simulink model "MPC_regul_real"  (R2017a)
settings: Solver=VariableStepAuto  StartTime=0.0  StopTime=40  RelTol=1e-3
values from neighbouring files (symbols this model uses):
  P_0 = eye(8)*100    [MPC_setup_nonlinear.m]    (also in sim_phi_ref.mat = [100 0 0 0 0 0 0 0 0 100 0 0 ... (64 elements, 8x8)]; sim_theta_ref.mat = [100 0 0 0 0 0 0 0 0 100 0 0 ... (64 elements, 8x8)])
  R1 = sqrtm(R)    [MPC_setup_nonlinear.m]    (also in sim_phi_ref.mat = [0.00081901538426  9.06300190075e-05; 9.06300190075e-05  0.0; sim_theta_ref.mat = [0.00081901538426  9.06300190075e-05; 9.06300190075e-05  0.0)
  Ts_control = 0.05    [MPC_setup_nonlinear.m]    (also in sim_phi_ref.mat = 0.02; sim_theta_ref.mat = 0.02)
  Ts_kalman = 0.01    [MPC_setup_nonlinear.m]    (also in sim_phi_ref.mat; sim_theta_ref.mat)
  x_0 = [0,-pi/4,0,0,0,0,0,0]    [MPC_setup_nonlinear.m]    (also in sim_phi_ref.mat = [0 -0.785398163397 0 0 0 0 0 0]; sim_theta_ref.mat = [0 -0.785398163397 0 0 0 0 0 0])
settings Model: Creator=sverreknutsen  LastModifiedBy=sverreknutsen
settings SolverCC: AlgebraicLoopSolver=LineSearch

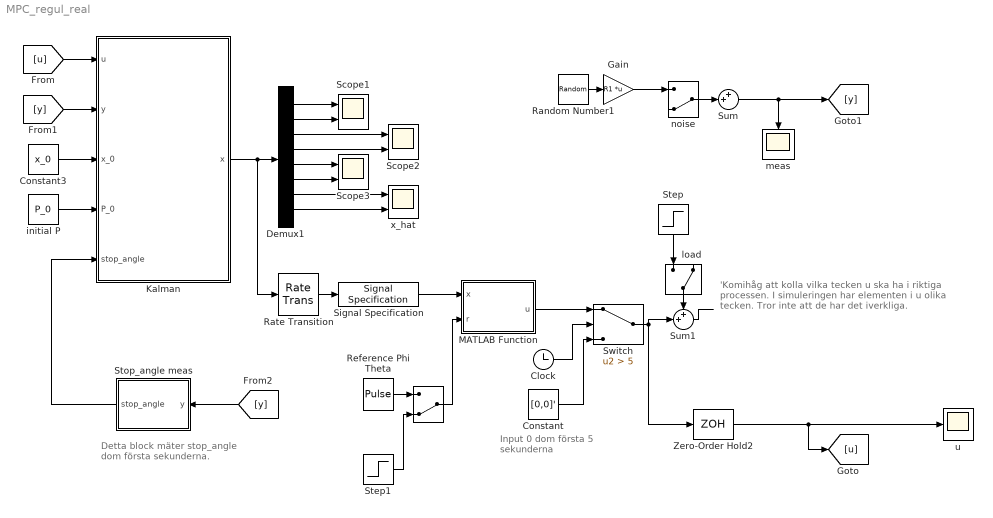
== system MPC_regul_real ==
  note: Input 0 dom första 5
      | sekunderna
  note: Detta block mäter stop_angle dom första sekunderna.
  note: 'Komihåg att kolla vilka tecken u ska ha i riktiga processen. I simuleringen har elementen i u olika tecken. Tror inte att de har det iverkliga.
  " " : ManualSwitch  CurrentSetting=0
  Clock : Clock
  Constant : Constant  Value=[0,0]'
  Constant3 : Constant  Value=x_0
  Demux1 : Demux  Outputs=8
  Gain : Gain  Gain=R1  Multiplication=Matrix(K*u)
  Kalman : MATLAB Function  TreatAsAtomicUnit=on
  MATLAB Function : MATLAB Function  TreatAsAtomicUnit=on
  Random Number1 : RandomNumber  Mean=[0,0]'  Variance=[1,1]'  Seed=[1,2]  SampleTime=Ts_kalman
  Rate Transition : RateTransition  X0=x_0  OutPortSampleTime=Ts_control
  "Reference Phi Theta " : DiscretePulseGenerator  PulseType=Time based  Amplitude=[-0.2,-pi/7]'  Period=10  PulseWidth=50
  Scope1 : Scope  NumInputPorts=2
  Scope2 : Scope  NumInputPorts=2
  Scope3 : Scope  NumInputPorts=2
  Signal Specification : SignalSpecification  Dimensions=[8 1]  SampleTime=Ts_control
  Step : Step  Time=30  Before=[0,0]'  After=[1,1]'*0.5  SampleTime=0
  Step1 : Step  Before=[0,0]'  After=[0,-pi/7]'  SampleTime=0
  Stop_angle meas : MATLAB Function  TreatAsAtomicUnit=on
  Sum : Sum  Inputs=++|
  Sum1 : Sum  Inputs=++|
  Switch : Switch  Criteria=u2 > Threshold  Threshold=5
  Zero-Order Hold2 : ZeroOrderHold  SampleTime=Ts_kalman
  "initial P " : Constant  Value=P_0
  "load " : ManualSwitch  CurrentSetting=0
  "meas " : Scope
  "noise " : ManualSwitch  CurrentSetting=0
  "u " : Scope
  "x_hat " : Scope  NumInputPorts=2
  wires:
  Signal Specification/1 -> MATLAB Function/1(x)
  Kalman/1(x) -> Demux1/1, Rate Transition/1
  Switch/1 -> Sum1/2, Zero-Order Hold2/1
  Constant/1 -> Switch/3
  "initial P "/1 -> Kalman/4(P_0)
  Constant3/1 -> Kalman/3(x_0)
  [u] -> Kalman/1(u)
  [y] -> Kalman/2(y)
  Rate Transition/1 -> Signal Specification/1
  Zero-Order Hold2/1 -> "u "/1, [u]
  Sum1/1 -> ?
  "load "/1 -> Sum1/1
  Step/1 -> "load "/1
  Clock/1 -> Switch/2
  MATLAB Function/1(u) -> Switch/1
  Demux1/8 -> "x_hat "/2
  Demux1/7 -> "x_hat "/1
  Demux1/1 -> Scope1/1
  Demux1/2 -> Scope1/2
  Demux1/3 -> Scope2/1
  Demux1/4 -> Scope2/2
  Sum/1 -> [y], "meas "/1
  Stop_angle meas/1(stop_angle) -> Kalman/5(stop_angle)
  Random Number1/1 -> Gain/1
  Gain/1 -> "noise "/1
  Demux1/5 -> Scope3/1
  Demux1/6 -> Scope3/2
  "noise "/1 -> Sum/2
  ? -> Sum/1
  [y] -> Stop_angle meas/1(y)
  "Reference Phi Theta "/1 -> " "/1
  " "/1 -> MATLAB Function/2(r)
  Step1/1 -> " "/2

== matlab function MPC_regul_real/Stop_angle meas ==
  data: y input; stop_angle output
function stop_angle = fcn(y)
x=y(2);
persistent i;
persistent x_;
if(isempty(i))
        i=0;
        x_=0;
end
    

   
    if(i<100)
    i=i+1;
    x_=x_+x;

    stop_angle=x_/i;
    else
      stop_angle=x_/i;
    end

== matlab function MPC_regul_real/MATLAB Function ==
  data: x input; u output; r input
function u = MPC(x,r)
%The MPC solver using CVXgen. 

coder.extrinsic('mycsolve'); %force simulink to accept that mycsolve will acctualy return u in a vector.
u = [0;0]; % pre-define u to be of correct type/size [u] = mycsolve(x);

% if(isempty(x)) %initialize
%     x=x_0;
%     u=mycsolve(x); %solve
% 
% else

    u=mycsolve(x,r); %solve
end

== matlab function MPC_regul_real/Kalman ==
  data: u input; x output; y input; x_0 input; P_0 input; stop_angle input
function x = extended_kalman(u,y,x_0,P_0,stop_angle)
persistent x_hat;
persistent P;
if(isempty(x_hat))
    x_hat=x_0;
    P=P_0;
end
coder.extrinsic('updateKalman');

[x_hat,P]=updateKalman(x_hat,u,y,P,stop_angle);
x=x_hat;
